simulink model "opt_SIRD"  (R2023a)
settings: Solver=VariableStepAuto  StartTime=0.0  StopTime=300  RelTol=1e-3
settings Model: Creator=Lawrence  LastModifiedBy=Lawrence

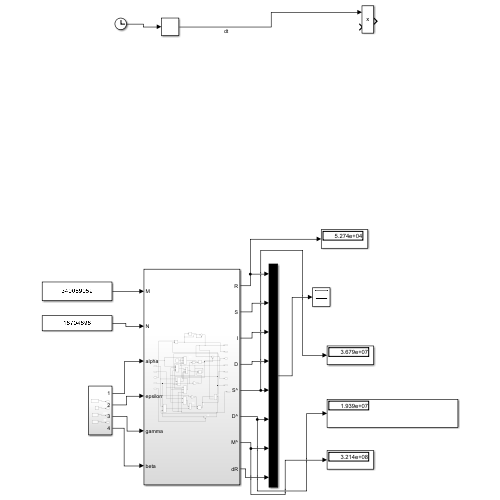
[thumbnail: Simulink's stored preview of the top-level diagram]
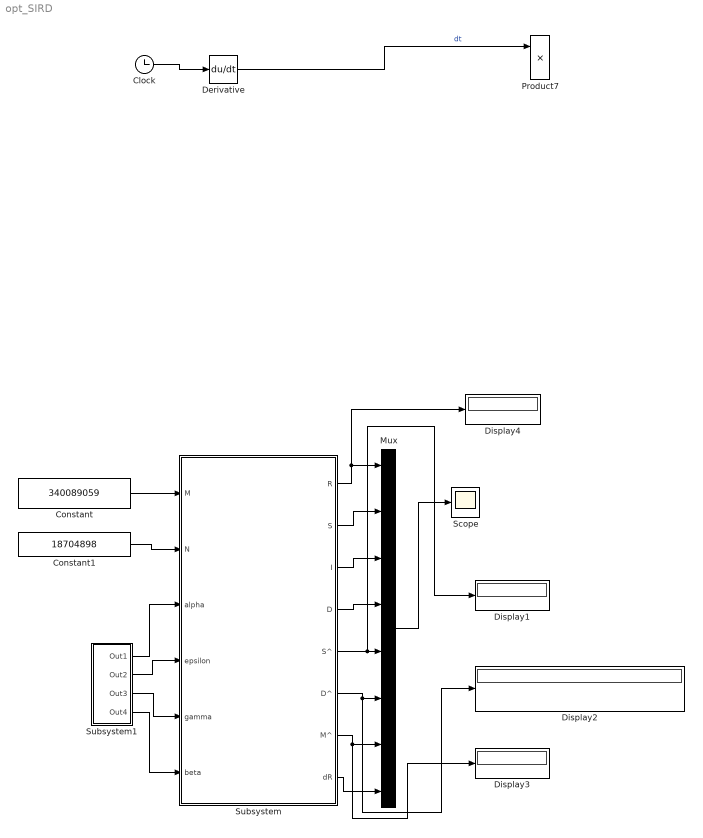
== system opt_SIRD ==
  Clock : Clock
  Constant : Constant  Value=340089059
  Constant1 : Constant  Value=18704898
  Derivative : Derivative
  Display{1..4} (4 alike) : Display
  Mux : Mux  Inputs=8
  Product7 : Product
  Scope : Scope
  Subsystem : Subsystem
  Subsystem1 : Subsystem
  wires:
  Clock/1 -> Derivative/1
  Derivative/1 -> Product7/1  "dt"
  Constant1/1 -> Subsystem/2(N)
  Constant/1 -> Subsystem/1(M)
  Subsystem/1(R) -> Display4/1, Mux/1
  Subsystem/2(S) -> Mux/2
  Subsystem/3(I) -> Mux/3
  Subsystem/4(D) -> Mux/4
  Subsystem/6(D^) -> Display2/1, Mux/6
  Subsystem/7(M^) -> Display3/1, Mux/7
  Subsystem/8(dR) -> Mux/8
  Mux/1 -> Scope/1
  Subsystem1/1(Out1) -> Subsystem/3(alpha)
  Subsystem1/2(Out2) -> Subsystem/4(epsilon)
  Subsystem1/3(Out3) -> Subsystem/5(gamma)
  Subsystem1/4(Out4) -> Subsystem/6(beta)
  Subsystem/5(S^) -> Display1/1, Mux/5

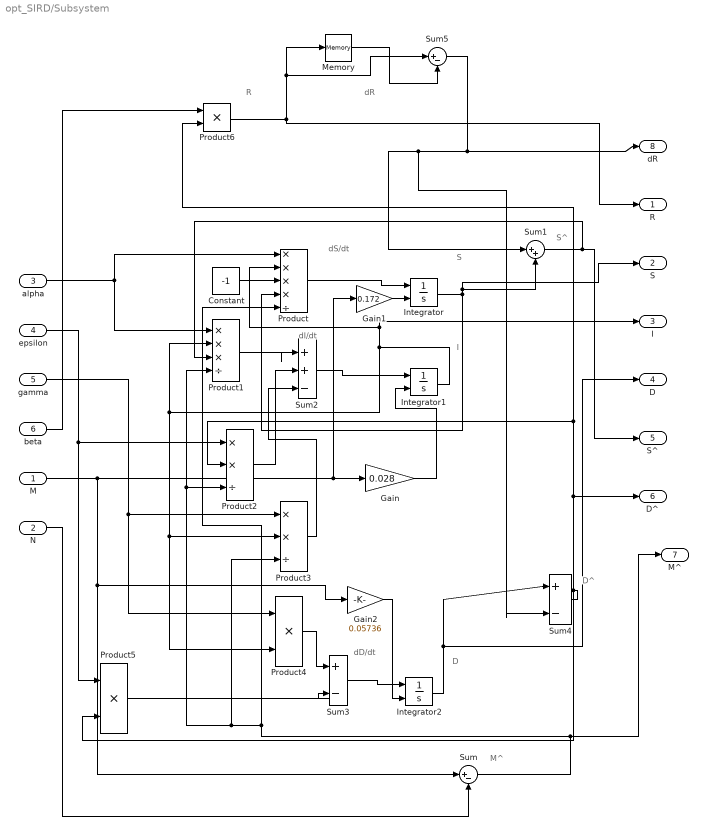
== system opt_SIRD/Subsystem ==
  note: M^
  note: S
  note: dS/dt
  note: dI/dt
  note: I
  note: dD/dt
  note: D
  note: dR
  note: R
  note: S^
  note: D^
  M : Inport
  N : Inport  Port=2
  alpha : Inport  Port=3
  epsilon : Inport  Port=4
  gamma : Inport  Port=5
  beta : Inport  Port=6
  Constant : Constant  Value=-1
  Gain : Gain  Gain=0.028
  Gain1 : Gain  Gain=0.172
  Gain2 : Gain  Gain=0.05736
  Integrator : Integrator  InitialConditionSource=external  InitialCondition=1000
  Integrator1 : Integrator  InitialConditionSource=external  InitialCondition=1000
  Integrator2 : Integrator  InitialConditionSource=external  InitialCondition=500
  Memory : Memory  LinearizeAsDelay=on
  Product : Product  Inputs=****/
  Product1 : Product  Inputs=***/
  Product2 : Product  Inputs=**/
  Product3 : Product  Inputs=**/
  Product4 : Product  Inputs=**
  Product5 : Product  Inputs=**
  Product6 : Product
  Sum{,3..5} (4 alike) : Sum  Inputs=|+-
  Sum1 : Sum  Inputs=|++
  Sum2 : Sum  Inputs=|++-
  R : Outport
  S : Outport  Port=2
  I : Outport  Port=3
  D : Outport  Port=4
  S^ : Outport  Port=5
  D^ : Outport  Port=6
  M^ : Outport  Port=7
  dR : Outport  Port=8
  wires:
  gamma/1 -> Product4/1, Product3/1
  M/1 -> Gain2/1, Sum/1, Gain/1, Gain1/1
  Product5/1 -> Sum3/2
  Product4/1 -> Sum3/1
  epsilon/1 -> Product5/1, Product2/1
  Integrator1/1 -> I/1, Product/2, Product4/2, Product3/2, Product1/2
  Product/1 -> Integrator/1
  N/1 -> Sum/2
  alpha/1 -> Product/1, Product1/1
  Product2/1 -> Sum2/2
  Sum/1 -> Product3/3, Product2/3, Product1/4, Product/5, M^/1
  Sum1/1 -> S^/1, Product1/3
  Product1/1 -> Sum2/1
  Constant/1 -> Product/3
  Sum5/1 -> Sum1/1, Sum4/2, dR/1
  Product6/1 -> Sum5/1, Memory/1, R/1
  Integrator/1 -> S/1, Sum1/2, Product/4
  Sum2/1 -> Integrator1/1
  Sum4/1 -> Product5/2, Product2/2, Product6/2, D^/1
  Product3/1 -> Sum2/3
  beta/1 -> Product6/1
  Sum3/1 -> Integrator2/1
  Integrator2/1 -> Sum4/1, D/1
  Memory/1 -> Sum5/2
  Gain/1 -> Integrator1/2
  Gain1/1 -> Integrator/2
  Gain2/1 -> Integrator2/2

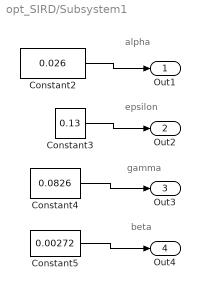
== system opt_SIRD/Subsystem1 ==
  note: beta
  note: gamma
  note: epsilon
  note: alpha
  Constant2 : Constant  Value=0.026
  Constant3 : Constant  Value=0.13
  Constant4 : Constant  Value=0.0826
  Constant5 : Constant  Value=0.00272
  Out1 : Outport
  Out2 : Outport  Port=2
  Out3 : Outport  Port=3
  Out4 : Outport  Port=4
  wires:
  Constant3/1 -> Out2/1
  Constant2/1 -> Out1/1
  Constant5/1 -> Out4/1
  Constant4/1 -> Out3/1
